simulink model "ClosedLoop_V1"  (R2021b)
settings: Solver=ode4  StartTime=0.0  StopTime=TMax  FixedStep=DT  MaxStep=DT  RelTol=1e-3  EnableMultiTasking=on
undefined symbols (not defined in the file or in its folder): CertificationSettings, Control, DiscIntNeverNeededParam, Drivetrain, OutList, P_InitAngle, RPM_Init, sigbuilder_block, SimConfig, strmatch
libraries: simulink_extras x4, simulink x1
(part 2 of 3)

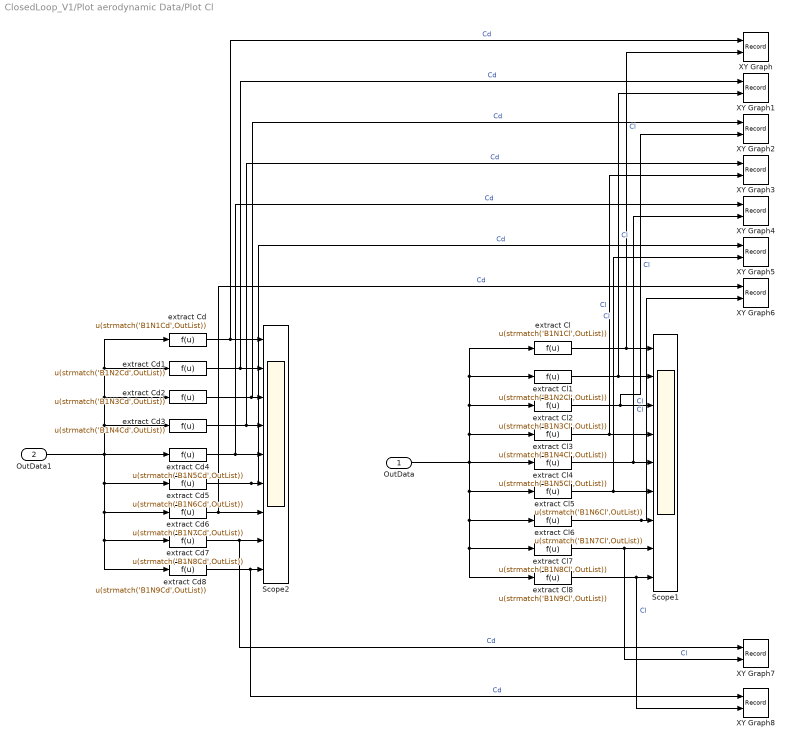
== system ClosedLoop_V1/Plot aerodynamic Data/Plot Cl ==
  OutData : Inport
  OutData1 : Inport  Port=2
  Scope1 : Scope  NumInputPorts=9
  Scope2 : Scope  NumInputPorts=9
  XY Graph : Record  FileSettingsInternal="{\"entries\":[{\"content\":{\"excelSettings\":{\"content\":{},\"type\":\"Streamout.ExcelSettings\"}},\"type\":\"Streamout.FileSettingStorage\",\"uuid\":\"b00f5487-2976-46a3-9d99-c10c1d8da87d\"}],\"packageUris\":[\"http://schema.mathworks.com/mf0/streamout_blocks/R2020a\"],\"version\":\"1.0\"}"  Layout=[1 1]  SignalsInternal="{\"entries\":[{\"content\":{\"signals\":[{\"content\":{\"blockPath\":[\"ClosedLoop_V1/Plot aerodynamic Data/Plot Cl/XY Graph\"],\"channel\":[],\"dimensions\":[1],\"domain\":\"ClosedLoop_V1/Plot aerodynamic Data/Plot Cl/XY Graph\",\"lineColor\":\"#a2142f\",\"plots\":[1],\"port\":1,\"sid\":[\"\"],\"signalID\":1325205,\"signalName\":\"Cd\"},\"type\":\"RecordBlkView.Signal\",\"uuid\":\"0eb759ee-437d-4b3f-a95d-ce2dedcb30b7\"},{\"content\":{\"blockPath\":[\"ClosedLoop_V1/Plot aerodynamic Data/Plot Cl/XY Graph\"],\"channel\":[],\"dimensions\":[1],\"domain\":\"ClosedLoop_V1/Plot aerodynamic Data/Plot Cl/XY Graph\",\"lineColor\":\"#139fff\",\"plots\":[1],\"port\":2,\"sid\":[\"\"],\"signalID\":1325209,\"signalName\":\"Cl\"},\"type\":\"RecordBlkView.Signal\",\"uuid\":\"04b02241-fa82-49a7-8999-ec9d8affa391\"}]},\"type\":\"RecordBlkView.InputSignals\",\"uuid\":\"daa39827-857a-4b2b-8609-f0bd73451858\"}],\"packageUris\":[\"http://schema.mathworks.com/mf0/streamout_blocks/R2020a\"],\"version\":\"1.0\"}"  VisualizationBindings="{\"xyplotplugin\":{\"info\":[{\"series\":[{\"bindingParametersList\":[{\"parameter\":\"X-Axis\",\"signalID\":1325205,\"signalName\":\"Cd\"},{\"parameter\":\"Y-Axis\",\"signalID\":1325209,\"signalName\":\"Cl\"}],\"seriesID\":63872}],\"subplotID\":1}]}}"  CompatibilityTag=XY  st=-1
  XY Graph1 : Record  FileSettingsInternal="{\"entries\":[{\"content\":{\"excelSettings\":{\"content\":{},\"type\":\"Streamout.ExcelSettings\"}},\"type\":\"Streamout.FileSettingStorage\",\"uuid\":\"94f4979b-c9e0-4134-9fa1-cf985e57c411\"}],\"packageUris\":[\"http://schema.mathworks.com/mf0/streamout_blocks/R2020a\"],\"version\":\"1.0\"}"  Layout=[1 1]  SignalsInternal="{\"entries\":[{\"content\":{\"signals\":[{\"content\":{\"blockPath\":[\"ClosedLoop_V1/Plot aerodynamic Data/Plot Cl/XY Graph1\"],\"channel\":[],\"dimensions\":[1],\"domain\":\"ClosedLoop_V1/Plot aerodynamic Data/Plot Cl/XY Graph1\",\"lineColor\":\"#a2142f\",\"plots\":[1],\"port\":1,\"sid\":[\"\"],\"signalID\":1325213,\"signalName\":\"Cd\"},\"type\":\"RecordBlkView.Signal\",\"uuid\":\"fcfc87ba-e672-4cf6-a8b9-8e6c01033c6e\"},{\"content\":{\"blockPath\":[\"ClosedLoop_V1/Plot aerodynamic Data/Plot Cl/XY Graph1\"],\"channel\":[],\"dimensions\":[1],\"domain\":\"ClosedLoop_V1/Plot aerodynamic Data/Plot Cl/XY Graph1\",\"lineColor\":\"#139fff\",\"plots\":[1],\"port\":2,\"sid\":[\"\"],\"signalID\":1325217,\"signalName\":\"Cl\"},\"type\":\"RecordBlkView.Signal\",\"uuid\":\"8be44a03-0071-4b23-8cb4-e834f8b4826c\"}]},\"type\":\"RecordBlkView.InputSignals\",\"uuid\":\"4f4c0f69-5f75-40c3-970b-0dcb076c4eae\"}],\"packageUris\":[\"http://schema.mathworks.com/mf0/streamout_blocks/R2020a\"],\"version\":\"1.0\"}"  VisualizationBindings="{\"xyplotplugin\":{\"info\":[{\"series\":[{\"bindingParametersList\":[{\"parameter\":\"X-Axis\",\"signalID\":1325213,\"signalName\":\"Cd\"},{\"parameter\":\"Y-Axis\",\"signalID\":1325217,\"signalName\":\"Cl\"}],\"seriesID\":24093}],\"subplotID\":1}]}}"  CompatibilityTag=XY  st=-1
  XY Graph2 : Record  FileSettingsInternal="{\"entries\":[{\"content\":{\"excelSettings\":{\"content\":{},\"type\":\"Streamout.ExcelSettings\"}},\"type\":\"Streamout.FileSettingStorage\",\"uuid\":\"4e5eaee2-b6a3-4246-9124-e66d8a1042dc\"}],\"packageUris\":[\"http://schema.mathworks.com/mf0/streamout_blocks/R2020a\"],\"version\":\"1.0\"}"  Layout=[1 1]  SignalsInternal="{\"entries\":[{\"content\":{\"signals\":[{\"content\":{\"blockPath\":[\"ClosedLoop_V1/Plot aerodynamic Data/Plot Cl/XY Graph2\"],\"channel\":[],\"dimensions\":[1],\"domain\":\"ClosedLoop_V1/Plot aerodynamic Data/Plot Cl/XY Graph2\",\"lineColor\":\"#a2142f\",\"plots\":[1],\"port\":1,\"sid\":[\"\"],\"signalID\":1325221,\"signalName\":\"Cd\"},\"type\":\"RecordBlkView.Signal\",\"uuid\":\"a1719d4d-a3ea-41e0-9451-246a2d23fc63\"},{\"content\":{\"blockPath\":[\"ClosedLoop_V1/Plot aerodynamic Data/Plot Cl/XY Graph2\"],\"channel\":[],\"dimensions\":[1],\"domain\":\"ClosedLoop_V1/Plot aerodynamic Data/Plot Cl/XY Graph2\",\"lineColor\":\"#139fff\",\"plots\":[1],\"port\":2,\"sid\":[\"\"],\"signalID\":1325225,\"signalName\":\"Cl\"},\"type\":\"RecordBlkView.Signal\",\"uuid\":\"30de273b-631d-455b-89d6-b0d743946a94\"}]},\"type\":\"RecordBlkView.InputSignals\",\"uuid\":\"fa155243-c94f-4b4c-8166-c767622a70d2\"}],\"packageUris\":[\"http://schema.mathworks.com/mf0/streamout_blocks/R2020a\"],\"version\":\"1.0\"}"  VisualizationBindings="{\"xyplotplugin\":{\"info\":[{\"series\":[{\"bindingParametersList\":[{\"parameter\":\"X-Axis\",\"signalID\":1325221,\"signalName\":\"Cd\"},{\"parameter\":\"Y-Axis\",\"signalID\":1325225,\"signalName\":\"Cl\"}],\"seriesID\":26258}],\"subplotID\":1}]}}"  CompatibilityTag=XY  st=-1
  XY Graph3 : Record  FileSettingsInternal="{\"entries\":[{\"content\":{\"excelSettings\":{\"content\":{},\"type\":\"Streamout.ExcelSettings\"}},\"type\":\"Streamout.FileSettingStorage\",\"uuid\":\"befbcad3-2241-43c1-98f9-6856619aad07\"}],\"packageUris\":[\"http://schema.mathworks.com/mf0/streamout_blocks/R2020a\"],\"version\":\"1.0\"}"  Layout=[1 1]  SignalsInternal="{\"entries\":[{\"content\":{\"signals\":[{\"content\":{\"blockPath\":[\"ClosedLoop_V1/Plot aerodynamic Data/Plot Cl/XY Graph3\"],\"channel\":[],\"dimensions\":[1],\"domain\":\"ClosedLoop_V1/Plot aerodynamic Data/Plot Cl/XY Graph3\",\"lineColor\":\"#a2142f\",\"plots\":[1],\"port\":1,\"sid\":[\"\"],\"signalID\":1325229,\"signalName\":\"Cd\"},\"type\":\"RecordBlkView.Signal\",\"uuid\":\"77f1f46a-23cf-4d3e-8ba2-b6f048b7fc30\"},{\"content\":{\"blockPath\":[\"ClosedLoop_V1/Plot aerodynamic Data/Plot Cl/XY Graph3\"],\"channel\":[],\"dimensions\":[1],\"domain\":\"ClosedLoop_V1/Plot aerodynamic Data/Plot Cl/XY Graph3\",\"lineColor\":\"#139fff\",\"plots\":[1],\"port\":2,\"sid\":[\"\"],\"signalID\":1325233,\"signalName\":\"Cl\"},\"type\":\"RecordBlkView.Signal\",\"uuid\":\"3d342543-18e3-42ba-a902-cf5380580f35\"}]},\"type\":\"RecordBlkView.InputSignals\",\"uuid\":\"aa93ef38-d005-41b7-956f-c3b12bea12ef\"}],\"packageUris\":[\"http://schema.mathworks.com/mf0/streamout_blocks/R2020a\"],\"version\":\"1.0\"}"  VisualizationBindings="{\"xyplotplugin\":{\"info\":[{\"series\":[{\"bindingParametersList\":[{\"parameter\":\"X-Axis\",\"signalID\":1325229,\"signalName\":\"Cd\"},{\"parameter\":\"Y-Axis\",\"signalID\":1325233,\"signalName\":\"Cl\"}],\"seriesID\":26014}],\"subplotID\":1}]}}"  CompatibilityTag=XY  st=-1
  XY Graph4 : Record  FileSettingsInternal="{\"entries\":[{\"content\":{\"excelSettings\":{\"content\":{},\"type\":\"Streamout.ExcelSettings\"}},\"type\":\"Streamout.FileSettingStorage\",\"uuid\":\"db6c0b38-0294-4e78-a363-89844ef9353c\"}],\"packageUris\":[\"http://schema.mathworks.com/mf0/streamout_blocks/R2020a\"],\"version\":\"1.0\"}"  Layout=[1 1]  SignalsInternal="{\"entries\":[{\"content\":{\"signals\":[{\"content\":{\"blockPath\":[\"ClosedLoop_V1/Plot aerodynamic Data/Plot Cl/XY Graph4\"],\"channel\":[],\"dimensions\":[1],\"domain\":\"ClosedLoop_V1/Plot aerodynamic Data/Plot Cl/XY Graph4\",\"lineColor\":\"#a2142f\",\"plots\":[1],\"port\":1,\"sid\":[\"\"],\"signalID\":1325237,\"signalName\":\"Cd\"},\"type\":\"RecordBlkView.Signal\",\"uuid\":\"0c91b63e-c937-4d51-adce-a1fbab03704b\"},{\"content\":{\"blockPath\":[\"ClosedLoop_V1/Plot aerodynamic Data/Plot Cl/XY Graph4\"],\"channel\":[],\"dimensions\":[1],\"domain\":\"ClosedLoop_V1/Plot aerodynamic Data/Plot Cl/XY Graph4\",\"lineColor\":\"#139fff\",\"plots\":[1],\"port\":2,\"sid\":[\"\"],\"signalID\":1325241,\"signalName\":\"Cl\"},\"type\":\"RecordBlkView.Signal\",\"uuid\":\"0b2e47cf-4e84-4860-af6a-48a2deb7a67a\"}]},\"type\":\"RecordBlkView.InputSignals\",\"uuid\":\"6ecca27e-ba54-49da-bcce-a4a3eb881ced\"}],\"packageUris\":[\"http://schema.mathworks.com/mf0/streamout_blocks/R2020a\"],\"version\":\"1.0\"}"  VisualizationBindings="{\"xyplotplugin\":{\"info\":[{\"series\":[{\"bindingParametersList\":[{\"parameter\":\"X-Axis\",\"signalID\":1325237,\"signalName\":\"Cd\"},{\"parameter\":\"Y-Axis\",\"signalID\":1325241,\"signalName\":\"Cl\"}],\"seriesID\":16519}],\"subplotID\":1}]}}"  CompatibilityTag=XY  st=-1
  XY Graph5 : Record  FileSettingsInternal="{\"entries\":[{\"content\":{\"excelSettings\":{\"content\":{},\"type\":\"Streamout.ExcelSettings\"}},\"type\":\"Streamout.FileSettingStorage\",\"uuid\":\"9460674a-7e25-40c0-b51d-5230c09c8e63\"}],\"packageUris\":[\"http://schema.mathworks.com/mf0/streamout_blocks/R2020a\"],\"version\":\"1.0\"}"  Layout=[1 1]  SignalsInternal="{\"entries\":[{\"content\":{\"signals\":[{\"content\":{\"blockPath\":[\"ClosedLoop_V1/Plot aerodynamic Data/Plot Cl/XY Graph5\"],\"channel\":[],\"dimensions\":[1],\"domain\":\"ClosedLoop_V1/Plot aerodynamic Data/Plot Cl/XY Graph5\",\"lineColor\":\"#a2142f\",\"plots\":[1],\"port\":1,\"sid\":[\"\"],\"signalID\":1325245,\"signalName\":\"Cd\"},\"type\":\"RecordBlkView.Signal\",\"uuid\":\"4c2cc2e6-f074-4467-ab2c-c656e1ab336f\"},{\"content\":{\"blockPath\":[\"ClosedLoop_V1/Plot aerodynamic Data/Plot Cl/XY Graph5\"],\"channel\":[],\"dimensions\":[1],\"domain\":\"ClosedLoop_V1/Plot aerodynamic Data/Plot Cl/XY Graph5\",\"lineColor\":\"#139fff\",\"plots\":[1],\"port\":2,\"sid\":[\"\"],\"signalID\":1325249,\"signalName\":\"Cl\"},\"type\":\"RecordBlkView.Signal\",\"uuid\":\"f16d4d46-7da3-4ca7-a621-15c7649c98ab\"}]},\"type\":\"RecordBlkView.InputSignals\",\"uuid\":\"8bb74b32-b33e-4f9b-9b24-77e9d0eb4d47\"}],\"packageUris\":[\"http://schema.mathworks.com/mf0/streamout_blocks/R2020a\"],\"version\":\"1.0\"}"  VisualizationBindings="{\"xyplotplugin\":{\"info\":[{\"series\":[{\"bindingParametersList\":[{\"parameter\":\"X-Axis\",\"signalID\":1325245,\"signalName\":\"Cd\"},{\"parameter\":\"Y-Axis\",\"signalID\":1325249,\"signalName\":\"Cl\"}],\"seriesID\":24904}],\"subplotID\":1}]}}"  CompatibilityTag=XY  st=-1
  XY Graph6 : Record  FileSettingsInternal="{\"entries\":[{\"content\":{\"excelSettings\":{\"content\":{},\"type\":\"Streamout.ExcelSettings\"}},\"type\":\"Streamout.FileSettingStorage\",\"uuid\":\"b7f41630-d128-4606-b5b0-76e3e016886f\"}],\"packageUris\":[\"http://schema.mathworks.com/mf0/streamout_blocks/R2020a\"],\"version\":\"1.0\"}"  Layout=[1 1]  SignalsInternal="{\"entries\":[{\"content\":{\"signals\":[{\"content\":{\"blockPath\":[\"ClosedLoop_V1/Plot aerodynamic Data/Plot Cl/XY Graph6\"],\"channel\":[],\"dimensions\":[1],\"domain\":\"ClosedLoop_V1/Plot aerodynamic Data/Plot Cl/XY Graph6\",\"lineColor\":\"#a2142f\",\"plots\":[1],\"port\":1,\"sid\":[\"\"],\"signalID\":1325253,\"signalName\":\"Cd\"},\"type\":\"RecordBlkView.Signal\",\"uuid\":\"3b1d38a9-1b72-4244-a152-a54677a825a9\"},{\"content\":{\"blockPath\":[\"ClosedLoop_V1/Plot aerodynamic Data/Plot Cl/XY Graph6\"],\"channel\":[],\"dimensions\":[1],\"domain\":\"ClosedLoop_V1/Plot aerodynamic Data/Plot Cl/XY Graph6\",\"lineColor\":\"#139fff\",\"plots\":[1],\"port\":2,\"sid\":[\"\"],\"signalID\":1325257,\"signalName\":\"Cl\"},\"type\":\"RecordBlkView.Signal\",\"uuid\":\"493a381b-ee0a-4854-92ec-9f5293569aef\"}]},\"type\":\"RecordBlkView.InputSignals\",\"uuid\":\"ecf3199d-e8dc-4fa5-af74-081fe56a48f2\"}],\"packageUris\":[\"http://schema.mathworks.com/mf0/streamout_blocks/R2020a\"],\"version\":\"1.0\"}"  VisualizationBindings="{\"xyplotplugin\":{\"info\":[{\"series\":[{\"bindingParametersList\":[{\"parameter\":\"X-Axis\",\"signalID\":1325253,\"signalName\":\"Cd\"},{\"parameter\":\"Y-Axis\",\"signalID\":1325257,\"signalName\":\"Cl\"}],\"seriesID\":438}],\"subplotID\":1}]}}"  CompatibilityTag=XY  st=-1
  XY Graph7 : Record  FileSettingsInternal="{\"entries\":[{\"content\":{\"excelSettings\":{\"content\":{},\"type\":\"Streamout.ExcelSettings\"}},\"type\":\"Streamout.FileSettingStorage\",\"uuid\":\"c9c28032-f02b-4770-9c4c-b7d50fb30e9d\"}],\"packageUris\":[\"http://schema.mathworks.com/mf0/streamout_blocks/R2020a\"],\"version\":\"1.0\"}"  Layout=[1 1]  SignalsInternal="{\"entries\":[{\"content\":{\"signals\":[{\"content\":{\"blockPath\":[\"ClosedLoop_V1/Plot aerodynamic Data/Plot Cl/XY Graph7\"],\"channel\":[],\"dimensions\":[1],\"domain\":\"ClosedLoop_V1/Plot aerodynamic Data/Plot Cl/XY Graph7\",\"lineColor\":\"#a2142f\",\"plots\":[1],\"port\":1,\"sid\":[\"\"],\"signalID\":1325261,\"signalName\":\"Cd\"},\"type\":\"RecordBlkView.Signal\",\"uuid\":\"4e0e9014-fb0a-41c8-a268-390f7d90f948\"},{\"content\":{\"blockPath\":[\"ClosedLoop_V1/Plot aerodynamic Data/Plot Cl/XY Graph7\"],\"channel\":[],\"dimensions\":[1],\"domain\":\"ClosedLoop_V1/Plot aerodynamic Data/Plot Cl/XY Graph7\",\"lineColor\":\"#139fff\",\"plots\":[1],\"port\":2,\"sid\":[\"\"],\"signalID\":1325265,\"signalName\":\"Cl\"},\"type\":\"RecordBlkView.Signal\",\"uuid\":\"ded6cb4d-91ec-4c24-91d7-1d6afa3da94f\"}]},\"type\":\"RecordBlkView.InputSignals\",\"uuid\":\"03fa7e92-1b0b-47ac-b291-5ef29a6e44e8\"}],\"packageUris\":[\"http://schema.mathworks.com/mf0/streamout_blocks/R2020a\"],\"version\":\"1.0\"}"  VisualizationBindings="{\"xyplotplugin\":{\"info\":[{\"series\":[{\"bindingParametersList\":[{\"parameter\":\"X-Axis\",\"signalID\":1325261,\"signalName\":\"Cd\"},{\"parameter\":\"Y-Axis\",\"signalID\":1325265,\"signalName\":\"Cl\"}],\"seriesID\":14437}],\"subplotID\":1}]}}"  CompatibilityTag=XY  st=-1
  XY Graph8 : Record  FileSettingsInternal="{\"entries\":[{\"content\":{\"excelSettings\":{\"content\":{},\"type\":\"Streamout.ExcelSettings\"}},\"type\":\"Streamout.FileSettingStorage\",\"uuid\":\"40722767-ecb4-45e0-a40b-ab64c3c9db6a\"}],\"packageUris\":[\"http://schema.mathworks.com/mf0/streamout_blocks/R2020a\"],\"version\":\"1.0\"}"  Layout=[1 1]  SignalsInternal="{\"entries\":[{\"content\":{\"signals\":[{\"content\":{\"blockPath\":[\"ClosedLoop_V1/Plot aerodynamic Data/Plot Cl/XY Graph8\"],\"channel\":[],\"dimensions\":[1],\"domain\":\"ClosedLoop_V1/Plot aerodynamic Data/Plot Cl/XY Graph8\",\"lineColor\":\"#a2142f\",\"plots\":[1],\"port\":1,\"sid\":[\"\"],\"signalID\":1325269,\"signalName\":\"Cd\"},\"type\":\"RecordBlkView.Signal\",\"uuid\":\"d84702cd-5f16-4f75-bbae-0c0931a26899\"},{\"content\":{\"blockPath\":[\"ClosedLoop_V1/Plot aerodynamic Data/Plot Cl/XY Graph8\"],\"channel\":[],\"dimensions\":[1],\"domain\":\"ClosedLoop_V1/Plot aerodynamic Data/Plot Cl/XY Graph8\",\"lineColor\":\"#139fff\",\"plots\":[1],\"port\":2,\"sid\":[\"\"],\"signalID\":1325273,\"signalName\":\"Cl\"},\"type\":\"RecordBlkView.Signal\",\"uuid\":\"e2c72b46-b8cd-45df-ac85-433b9a479b8a\"}]},\"type\":\"RecordBlkView.InputSignals\",\"uuid\":\"495dfdb2-5976-4d9a-9394-6b3494943b23\"}],\"packageUris\":[\"http://schema.mathworks.com/mf0/streamout_blocks/R2020a\"],\"version\":\"1.0\"}"  VisualizationBindings="{\"xyplotplugin\":{\"info\":[{\"series\":[{\"bindingParametersList\":[{\"parameter\":\"X-Axis\",\"signalID\":1325269,\"signalName\":\"Cd\"},{\"parameter\":\"Y-Axis\",\"signalID\":1325273,\"signalName\":\"Cl\"}],\"seriesID\":44046}],\"subplotID\":1}]}}"  CompatibilityTag=XY  st=-1
  extract Cd : Fcn  Expr=u(strmatch('B1N1Cd',OutList))
  extract Cd1 : Fcn  Expr=u(strmatch('B1N2Cd',OutList))
  extract Cd2 : Fcn  Expr=u(strmatch('B1N3Cd',OutList))
  extract Cd3 : Fcn  Expr=u(strmatch('B1N4Cd',OutList))
  extract Cd4 : Fcn  Expr=u(strmatch('B1N5Cd',OutList))
  extract Cd5 : Fcn  Expr=u(strmatch('B1N6Cd',OutList))
  extract Cd6 : Fcn  Expr=u(strmatch('B1N7Cd',OutList))
  extract Cd7 : Fcn  Expr=u(strmatch('B1N8Cd',OutList))
  extract Cd8 : Fcn  Expr=u(strmatch('B1N9Cd',OutList))
  extract Cl : Fcn  Expr=u(strmatch('B1N1Cl',OutList))
  extract Cl1 : Fcn  Expr=u(strmatch('B1N2Cl',OutList))
  extract Cl2 : Fcn  Expr=u(strmatch('B1N3Cl',OutList))
  extract Cl3 : Fcn  Expr=u(strmatch('B1N4Cl',OutList))
  extract Cl4 : Fcn  Expr=u(strmatch('B1N5Cl',OutList))
  extract Cl5 : Fcn  Expr=u(strmatch('B1N6Cl',OutList))
  extract Cl6 : Fcn  Expr=u(strmatch('B1N7Cl',OutList))
  extract Cl7 : Fcn  Expr=u(strmatch('B1N8Cl',OutList))
  extract Cl8 : Fcn  Expr=u(strmatch('B1N9Cl',OutList))
  wires:
  OutData/1 -> extract Cl/1, extract Cl1/1, extract Cl2/1, extract Cl3/1, extract Cl4/1, extract Cl5/1, extract Cl6/1, extract Cl8/1, extract Cl7/1
  extract Cl/1 -> XY Graph/2, Scope1/1  "Cl"
  extract Cl1/1 -> XY Graph1/2, Scope1/2  "Cl"
  extract Cl2/1 -> XY Graph2/2, Scope1/3  "Cl"
  extract Cl3/1 -> XY Graph3/2, Scope1/4  "Cl"
  extract Cl4/1 -> XY Graph4/2, Scope1/5  "Cl"
  extract Cl5/1 -> XY Graph5/2, Scope1/6  "Cl"
  extract Cl6/1 -> XY Graph6/2, Scope1/7  "Cl"
  extract Cl7/1 -> XY Graph7/2, Scope1/8  "Cl"
  extract Cl8/1 -> XY Graph8/2, Scope1/9  "Cl"
  extract Cd2/1 -> XY Graph2/1, Scope2/3  "Cd"
  extract Cd8/1 -> XY Graph8/1, Scope2/9  "Cd"
  extract Cd4/1 -> XY Graph4/1, Scope2/5  "Cd"
  extract Cd3/1 -> XY Graph3/1, Scope2/4  "Cd"
  extract Cd/1 -> XY Graph/1, Scope2/1  "Cd"
  OutData1/1 -> extract Cd4/1, extract Cd5/1, extract Cd6/1, extract Cd8/1, extract Cd7/1, extract Cd3/1, extract Cd2/1, extract Cd1/1, extract Cd/1
  extract Cd1/1 -> XY Graph1/1, Scope2/2  "Cd"
  extract Cd7/1 -> XY Graph7/1, Scope2/8  "Cd"
  extract Cd5/1 -> XY Graph5/1, Scope2/6  "Cd"
  extract Cd6/1 -> Scope2/7, XY Graph6/1  "Cd"

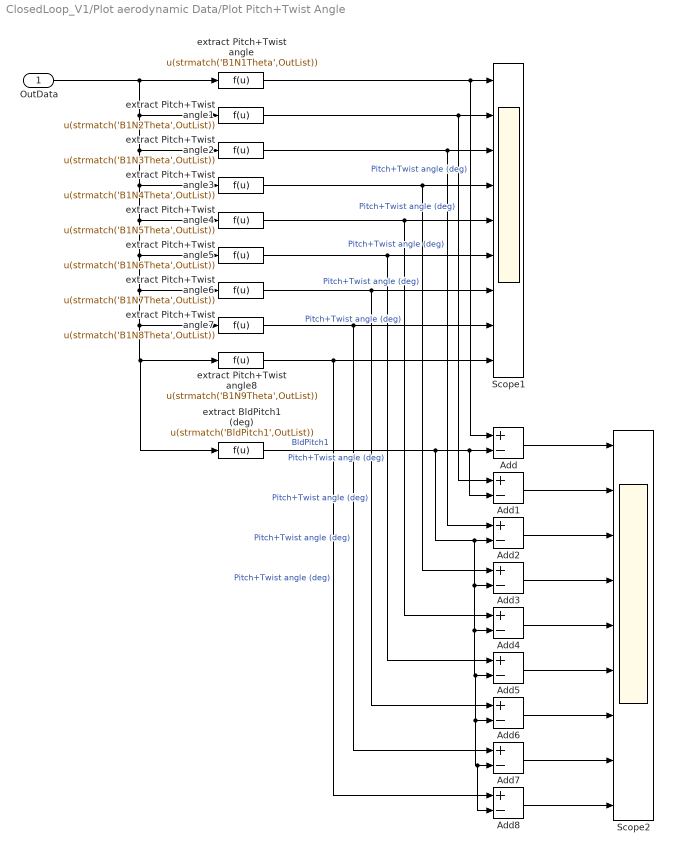
== system ClosedLoop_V1/Plot aerodynamic Data/Plot Pitch+Twist Angle ==
  OutData : Inport
  Add{,1..8} (9 alike) : Sum  Inputs=+-
  Scope1 : Scope  NumInputPorts=9
  Scope2 : Scope  NumInputPorts=9
  extract BldPitch1 (deg) : Fcn  Expr=u(strmatch('BldPitch1',OutList))
  extract Pitch+Twist angle : Fcn  Expr=u(strmatch('B1N1Theta',OutList))
  extract Pitch+Twist angle1 : Fcn  Expr=u(strmatch('B1N2Theta',OutList))
  extract Pitch+Twist angle2 : Fcn  Expr=u(strmatch('B1N3Theta',OutList))
  extract Pitch+Twist angle3 : Fcn  Expr=u(strmatch('B1N4Theta',OutList))
  extract Pitch+Twist angle4 : Fcn  Expr=u(strmatch('B1N5Theta',OutList))
  extract Pitch+Twist angle5 : Fcn  Expr=u(strmatch('B1N6Theta',OutList))
  extract Pitch+Twist angle6 : Fcn  Expr=u(strmatch('B1N7Theta',OutList))
  extract Pitch+Twist angle7 : Fcn  Expr=u(strmatch('B1N8Theta',OutList))
  extract Pitch+Twist angle8 : Fcn  Expr=u(strmatch('B1N9Theta',OutList))
  wires:
  extract Pitch+Twist angle/1 -> Add/1, Scope1/1  "Pitch+Twist angle (deg)"
  OutData/1 -> extract Pitch+Twist angle/1, extract Pitch+Twist angle1/1, extract Pitch+Twist angle2/1, extract Pitch+Twist angle3/1, extract Pitch+Twist angle4/1, extract Pitch+Twist angle5/1, extract Pitch+Twist angle6/1, extract BldPitch1 (deg)/1, extract Pitch+Twist angle8/1, extract Pitch+Twist angle7/1
  extract Pitch+Twist angle1/1 -> Add1/1, Scope1/2  "Pitch+Twist angle (deg)"
  extract Pitch+Twist angle2/1 -> Add2/1, Scope1/3  "Pitch+Twist angle (deg)"
  extract Pitch+Twist angle3/1 -> Add3/1, Scope1/4  "Pitch+Twist angle (deg)"
  extract Pitch+Twist angle4/1 -> Add4/1, Scope1/5  "Pitch+Twist angle (deg)"
  extract Pitch+Twist angle5/1 -> Add5/1, Scope1/6  "Pitch+Twist angle (deg)"
  extract Pitch+Twist angle6/1 -> Add6/1, Scope1/7  "Pitch+Twist angle (deg)"
  extract Pitch+Twist angle7/1 -> Add7/1, Scope1/8  "Pitch+Twist angle (deg)"
  extract Pitch+Twist angle8/1 -> Add8/1, Scope1/9  "Pitch+Twist angle (deg)"
  extract BldPitch1 (deg)/1 -> Add8/2, Add7/2, Add6/2, Add5/2, Add4/2, Add3/2, Add2/2, Add1/2, Add/2  "BldPitch1"
  Add/1 -> Scope2/1
  Add1/1 -> Scope2/2
  Add2/1 -> Scope2/3
  Add3/1 -> Scope2/4
  Add4/1 -> Scope2/5
  Add5/1 -> Scope2/6
  Add6/1 -> Scope2/7
  Add7/1 -> Scope2/8
  Add8/1 -> Scope2/9

== system ClosedLoop_V1/Plot aerodynamic Data/Plot Reynolds number ==
  note: B1N1Re      Reynolds number (in millions) at Blade 1, Node 1
      | B1N2Re      Reynolds number (in millions) at Blade 1, Node 2
      | B1N3Re      Reynolds number (in millions) at Blade 1, Node 3
      | B1N4Re      Reynolds number (in millions) at Blade 1, Node 4
      | B1N5Re      Reynolds number (in millions) at Blade 1, Node 5
      | B1N6Re      Reynolds number (in millions) at Blade 1, Node 6
      | B1N7Re      Reynolds number (in millions) at Blade 1, Node 7
      | B1N8Re      Reynolds number (in millions) at Blade 1, Node 8
      | B1N9Re      Reynolds number (in millions) at Blade 1, Node 9
  OutData1 : Inport
  Scope : Scope  NumInputPorts=9
  "extract Reynolds number (in millions) at Blade 1, Node 1" : Fcn  Expr=u(strmatch('B1N1Re',OutList))
  "extract Reynolds number (in millions) at Blade 1, Node 2" : Fcn  Expr=u(strmatch('B1N2Re',OutList))
  "extract Reynolds number (in millions) at Blade 1, Node 3" : Fcn  Expr=u(strmatch('B1N3Re',OutList))
  "extract Reynolds number (in millions) at Blade 1, Node 4" : Fcn  Expr=u(strmatch('B1N4Re',OutList))
  "extract Reynolds number (in millions) at Blade 1, Node 5" : Fcn  Expr=u(strmatch('B1N5Re',OutList))
  "extract Reynolds number (in millions) at Blade 1, Node 6" : Fcn  Expr=u(strmatch('B1N6Re',OutList))
  "extract Reynolds number (in millions) at Blade 1, Node 7" : Fcn  Expr=u(strmatch('B1N7Re',OutList))
  "extract Reynolds number (in millions) at Blade 1, Node 8" : Fcn  Expr=u(strmatch('B1N8Re',OutList))
  "extract Reynolds number (in millions) at Blade 1, Node 9" : Fcn  Expr=u(strmatch('B1N9Re',OutList))
  wires:
  OutData1/1 -> "extract Reynolds number (in millions) at Blade 1, Node 9"/1, "extract Reynolds number (in millions) at Blade 1, Node 8"/1, "extract Reynolds number (in millions) at Blade 1, Node 7"/1, "extract Reynolds number (in millions) at Blade 1, Node 6"/1, "extract Reynolds number (in millions) at Blade 1, Node 5"/1, "extract Reynolds number (in millions) at Blade 1, Node 4"/1, "extract Reynolds number (in millions) at Blade 1, Node 3"/1, "extract Reynolds number (in millions) at Blade 1, Node 2"/1, "extract Reynolds number (in millions) at Blade 1, Node 1"/1
  "extract Reynolds number (in millions) at Blade 1, Node 8"/1 -> Scope/8  "Reynolds number (in millions) at Blade 1, Node 8"
  "extract Reynolds number (in millions) at Blade 1, Node 3"/1 -> Scope/3  "Reynolds number (in millions) at Blade 1, Node 3"
  "extract Reynolds number (in millions) at Blade 1, Node 5"/1 -> Scope/5  "Reynolds number (in millions) at Blade 1, Node 5"
  "extract Reynolds number (in millions) at Blade 1, Node 7"/1 -> Scope/7  "Reynolds number (in millions) at Blade 1, Node 7"
  "extract Reynolds number (in millions) at Blade 1, Node 1"/1 -> Scope/1  "Reynolds number (in millions) at Blade 1, Node 1"
  "extract Reynolds number (in millions) at Blade 1, Node 6"/1 -> Scope/6  "Reynolds number (in millions) at Blade 1, Node 6"
  "extract Reynolds number (in millions) at Blade 1, Node 4"/1 -> Scope/4  "Reynolds number (in millions) at Blade 1, Node 4"
  "extract Reynolds number (in millions) at Blade 1, Node 9"/1 -> Scope/9  "Reynolds number (in millions) at Blade 1, Node 9"
  "extract Reynolds number (in millions) at Blade 1, Node 2"/1 -> Scope/2  "Reynolds number (in millions) at Blade 1, Node 2"

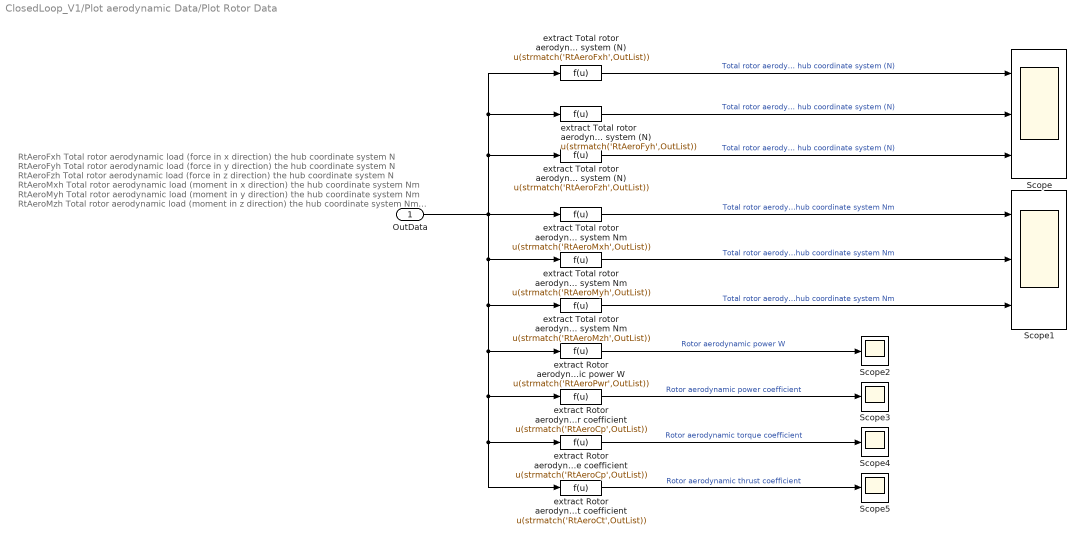
== system ClosedLoop_V1/Plot aerodynamic Data/Plot Rotor Data ==
  note: RtAeroFxh   Total rotor aerodynamic load (force in x direction) the hub coordinate system N
      | RtAeroFyh   Total rotor aerodynamic load (force in y direction) the hub coordinate system N
      | RtAeroFzh   Total rotor aerodynamic load (force in z direction) the hub coordinate system N
      | RtAeroMxh   Total rotor aerodynamic load (moment in x direction) the hub coordinate system Nm
      | RtAeroMyh   Total rotor aerodynamic load (moment in y direction) the hub coordinate system Nm
      | RtAeroMzh   Total rotor aerodynamic load (moment in z direction) the hub coordinate system Nm
      | RtAeroPwr   Rotor aerodynamic power W
      | RtAeroCp    Rotor aerodynamic power coefficient
      | RtAeroCq    Rotor aerodynamic torque coefficient
      | RtAeroCt    Rotor aerodynamic thrust coefficient
  OutData : Inport
  Scope : Scope  NumInputPorts=3
  Scope1 : Scope  NumInputPorts=3
  Scope{2..5} (4 alike) : Scope
  extract Rotor aerodynamic power W : Fcn  Expr=u(strmatch('RtAeroPwr',OutList))
  extract Rotor aerodynamic power coefficient : Fcn  Expr=u(strmatch('RtAeroCp',OutList))
  extract Rotor aerodynamic thrust coefficient : Fcn  Expr=u(strmatch('RtAeroCt',OutList))
  extract Rotor aerodynamic torque coefficient : Fcn  Expr=u(strmatch('RtAeroCp',OutList))
  extract Total rotor aerodynamic load (force in x direction) hub coordinate system (N) : Fcn  Expr=u(strmatch('RtAeroFxh',OutList))
  extract Total rotor aerodynamic load (force in y direction) hub coordinate system (N) : Fcn  Expr=u(strmatch('RtAeroFyh',OutList))
  extract Total rotor aerodynamic load (force in z direction) hub coordinate system (N) : Fcn  Expr=u(strmatch('RtAeroFzh',OutList))
  extract Total rotor aerodynamic load (moment in x direction) the hub coordinate system Nm : Fcn  Expr=u(strmatch('RtAeroMxh',OutList))
  extract Total rotor aerodynamic load (moment in y direction) the hub coordinate system Nm : Fcn  Expr=u(strmatch('RtAeroMyh',OutList))
  extract Total rotor aerodynamic load (moment in z direction) the hub coordinate system Nm : Fcn  Expr=u(strmatch('RtAeroMzh',OutList))
  wires:
  extract Total rotor aerodynamic load (force in x direction) hub coordinate system (N)/1 -> Scope/1  "Total rotor aerodynamic load (force in x direction) hub coordinate system (N)"
  OutData/1 -> extract Rotor aerodynamic thrust coefficient/1, extract Rotor aerodynamic torque coefficient/1, extract Rotor aerodynamic power coefficient/1, extract Rotor aerodynamic power W/1, extract Total rotor aerodynamic load (moment in z direction) the hub coordinate system Nm/1, extract Total rotor aerodynamic load (moment in y direction) the hub coordinate system Nm/1, extract Total rotor aerodynamic load (force in z direction) hub coordinate system (N)/1, extract Total rotor aerodynamic load (force in y direction) hub coordinate system (N)/1, extract Total rotor aerodynamic load (force in x direction) hub coordinate system (N)/1, extract Total rotor aerodynamic load (moment in x direction) the hub coordinate system Nm/1
  extract Total rotor aerodynamic load (force in y direction) hub coordinate system (N)/1 -> Scope/2  "Total rotor aerodynamic load (force in y direction) hub coordinate system (N)"
  extract Total rotor aerodynamic load (force in z direction) hub coordinate system (N)/1 -> Scope/3  "Total rotor aerodynamic load (force in z direction) hub coordinate system (N)"
  extract Total rotor aerodynamic load (moment in x direction) the hub coordinate system Nm/1 -> Scope1/1  "Total rotor aerodynamic load (moment in x direction) the hub coordinate system Nm"
  extract Total rotor aerodynamic load (moment in y direction) the hub coordinate system Nm/1 -> Scope1/2  "Total rotor aerodynamic load (moment in y direction) the hub coordinate system Nm"
  extract Total rotor aerodynamic load (moment in z direction) the hub coordinate system Nm/1 -> Scope1/3  "Total rotor aerodynamic load (moment in z direction) the hub coordinate system Nm"
  extract Rotor aerodynamic power W/1 -> Scope2/1  "Rotor aerodynamic power W"
  extract Rotor aerodynamic power coefficient/1 -> Scope3/1  "Rotor aerodynamic power coefficient"
  extract Rotor aerodynamic torque coefficient/1 -> Scope4/1  "Rotor aerodynamic torque coefficient"
  extract Rotor aerodynamic thrust coefficient/1 -> Scope5/1  "Rotor aerodynamic thrust coefficient"

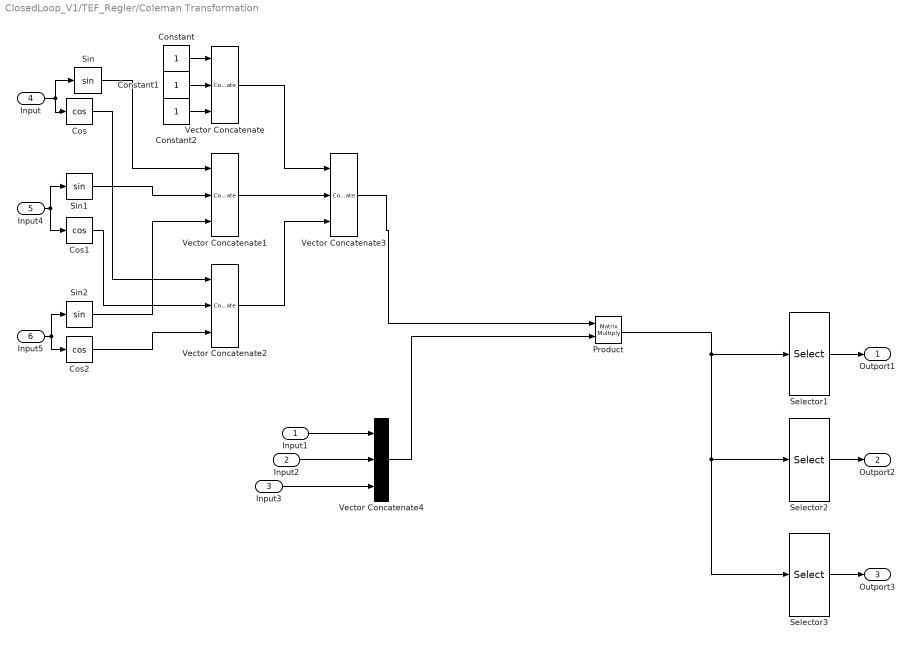
== system ClosedLoop_V1/TEF_Regler/Coleman Transformation ==
  Input1 : Inport
  Input2 : Inport  Port=2
  Input3 : Inport  Port=3
  Input : Inport  Port=4
  Input4 : Inport  Port=5
  Input5 : Inport  Port=6
  Constant : Constant
  Constant1 : Constant
  Constant2 : Constant
  Cos : Trigonometry  Operator=cos
  Cos1 : Trigonometry  Operator=cos
  Cos2 : Trigonometry  Operator=cos
  Product : Product  Multiplication=Matrix(*)
  Selector1 : Selector  InputPortWidth=3  IndexOptions=Index vector (dialog)  Indices=[1]  OutputSizes=1
  Selector2 : Selector  InputPortWidth=3  IndexOptions=Index vector (dialog)  Indices=[2]  OutputSizes=1
  Selector3 : Selector  InputPortWidth=3  IndexOptions=Index vector (dialog)  Indices=[3]  OutputSizes=1
  Sin : Trigonometry
  Sin1 : Trigonometry
  Sin2 : Trigonometry
  Vector Concatenate{,1..2,4} (4 alike) : Concatenate  NumInputs=3
  Vector Concatenate3 : Concatenate  NumInputs=3  Mode=Multidimensional array  ConcatenateDimension=2
  Outport1 : Outport  VectorParamsAs1DForOutWhenUnconnected=off
  Outport2 : Outport  Port=2  VectorParamsAs1DForOutWhenUnconnected=off
  Outport3 : Outport  Port=3  VectorParamsAs1DForOutWhenUnconnected=off
  wires:
  Vector Concatenate/1 -> Vector Concatenate3/1
  Product/1 -> Selector3/1, Selector2/1, Selector1/1
  Input/1 -> Cos/1, Sin/1
  Sin/1 -> Vector Concatenate1/1
  Cos2/1 -> Vector Concatenate2/3
  Sin1/1 -> Vector Concatenate1/2
  Cos/1 -> Vector Concatenate2/1
  Cos1/1 -> Vector Concatenate2/2
  Sin2/1 -> Vector Concatenate1/3
  Constant1/1 -> Vector Concatenate/2
  Constant/1 -> Vector Concatenate/1
  Input5/1 -> Cos2/1, Sin2/1
  Vector Concatenate1/1 -> Vector Concatenate3/2
  Vector Concatenate4/1 -> Product/2
  Selector1/1 -> Outport1/1
  Selector2/1 -> Outport2/1
  Selector3/1 -> Outport3/1
  Vector Concatenate2/1 -> Vector Concatenate3/3
  Input4/1 -> Cos1/1, Sin1/1
  Vector Concatenate3/1 -> Product/1
  Constant2/1 -> Vector Concatenate/3
  Input1/1 -> Vector Concatenate4/1
  Input2/1 -> Vector Concatenate4/2
  Input3/1 -> Vector Concatenate4/3

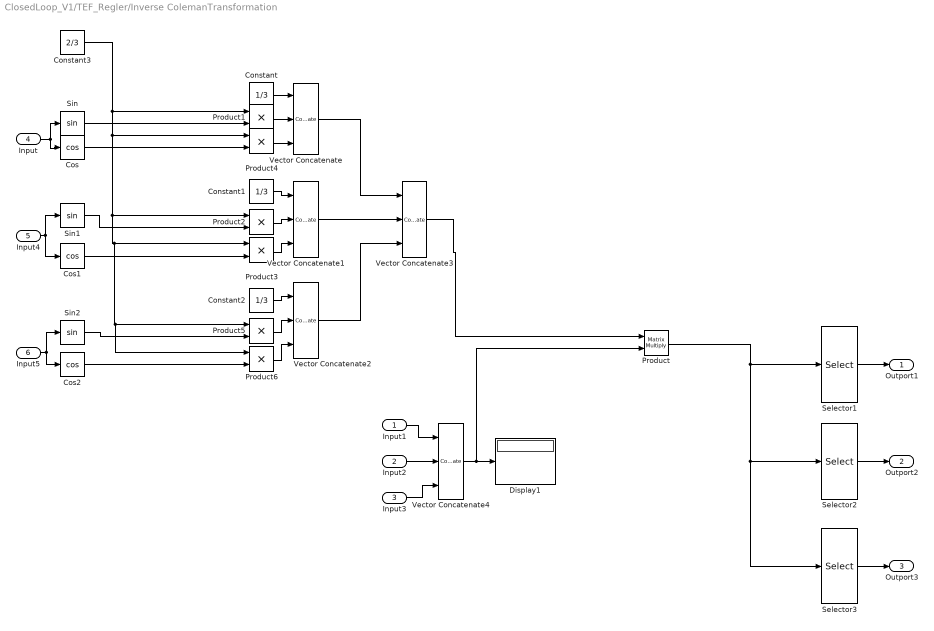
== system ClosedLoop_V1/TEF_Regler/Inverse ColemanTransformation ==
  Input1 : Inport
  Input2 : Inport  Port=2
  Input3 : Inport  Port=3
  Input : Inport  Port=4
  Input4 : Inport  Port=5
  Input5 : Inport  Port=6
  Constant : Constant  Value=1/3
  Constant1 : Constant  Value=1/3
  Constant2 : Constant  Value=1/3
  Constant3 : Constant  Value=2/3
  Cos : Trigonometry  Operator=cos
  Cos1 : Trigonometry  Operator=cos
  Cos2 : Trigonometry  Operator=cos
  Display1 : Display
  Product : Product  Multiplication=Matrix(*)
  Product{1..6} (6 alike) : Product
  Selector1 : Selector  InputPortWidth=3  IndexOptions=Index vector (dialog)  Indices=[1]  OutputSizes=1
  Selector2 : Selector  InputPortWidth=3  IndexOptions=Index vector (dialog)  Indices=[2]  OutputSizes=1
  Selector3 : Selector  InputPortWidth=3  IndexOptions=Index vector (dialog)  Indices=[3]  OutputSizes=1
  Sin : Trigonometry
  Sin1 : Trigonometry
  Sin2 : Trigonometry
  Vector Concatenate{,1..2,4} (4 alike) : Concatenate  NumInputs=3  Mode=Multidimensional array
  Vector Concatenate3 : Concatenate  NumInputs=3  Mode=Multidimensional array  ConcatenateDimension=2
  Outport1 : Outport  VectorParamsAs1DForOutWhenUnconnected=off
  Outport2 : Outport  Port=2  VectorParamsAs1DForOutWhenUnconnected=off
  Outport3 : Outport  Port=3  VectorParamsAs1DForOutWhenUnconnected=off
  wires:
  Cos2/1 -> Product6/2
  Sin2/1 -> Product5/2
  Cos1/1 -> Product3/2
  Cos/1 -> Product4/2
  Constant3/1 -> Product6/1, Product5/1, Product3/1, Product2/1, Product4/1, Product1/1
  Input2/1 -> Vector Concatenate4/2
  Input1/1 -> Vector Concatenate4/1
  Vector Concatenate4/1 -> Product/2, Display1/1
  Input3/1 -> Vector Concatenate4/3
  Product5/1 -> Vector Concatenate2/2
  Sin/1 -> Product1/2
  Product3/1 -> Vector Concatenate1/3
  Constant2/1 -> Vector Concatenate2/1
  Product6/1 -> Vector Concatenate2/3
  Constant1/1 -> Vector Concatenate1/1
  Sin1/1 -> Product2/2
  Product4/1 -> Vector Concatenate/3
  Input5/1 -> Cos2/1, Sin2/1
  Vector Concatenate3/1 -> Product/1
  Vector Concatenate/1 -> Vector Concatenate3/1
  Input/1 -> Sin/1, Cos/1
  Vector Concatenate2/1 -> Vector Concatenate3/3
  Vector Concatenate1/1 -> Vector Concatenate3/2
  Constant/1 -> Vector Concatenate/1
  Product1/1 -> Vector Concatenate/2
  Product2/1 -> Vector Concatenate1/2
  Input4/1 -> Cos1/1, Sin1/1
  Selector1/1 -> Outport1/1
  Product/1 -> Selector3/1, Selector2/1, Selector1/1
  Selector3/1 -> Outport3/1
  Selector2/1 -> Outport2/1

== system ClosedLoop_V1/TEF_Regler/Subsystem ==
  In1 : Inport
  Derivative : Derivative
  Gain : Gain  Gain=SimConfig.controller.TEF.K_P
  Gain1 : Gain  Gain=SimConfig.controller.TEF.K_I
  Gain2 : Gain  Gain=SimConfig.controller.TEF.K_D
  Integrator : Integrator
  Scope : Scope  NumInputPorts=2
  Scope1 : Scope  NumInputPorts=2
  Scope2 : Scope  NumInputPorts=5
  Sum : Sum  Inputs=+++
  Out1 : Outport  VectorParamsAs1DForOutWhenUnconnected=off
  wires:
  Sum/1 -> Scope2/4, Out1/1
  Integrator/1 -> Gain1/1  "I"
  Derivative/1 -> Gain2/1
  In1/1 -> Scope2/5, Scope/1, Gain/1, Scope1/2, Integrator/1, Derivative/1
  Gain/1 -> Scope/2, Scope2/2, Sum/2  "P"
  Gain1/1 -> Scope1/1, Scope2/3, Sum/3
  Gain2/1 -> Sum/1, Scope2/1  "D"

== system ClosedLoop_V1/TEF_Regler/Subsystem1 ==
  In1 : Inport
  Derivative : Derivative
  Gain : Gain  Gain=SimConfig.controller.TEF.K_P
  Gain1 : Gain  Gain=SimConfig.controller.TEF.K_I
  Gain2 : Gain  Gain=SimConfig.controller.TEF.K_D
  Integrator : Integrator
  Sum : Sum  Inputs=+++
  Out1 : Outport  VectorParamsAs1DForOutWhenUnconnected=off
  wires:
  Gain2/1 -> Sum/1
  Gain1/1 -> Sum/3
  Gain/1 -> Sum/2
  In1/1 -> Derivative/1, Integrator/1, Gain/1
  Derivative/1 -> Gain2/1
  Integrator/1 -> Gain1/1
  Sum/1 -> Out1/1

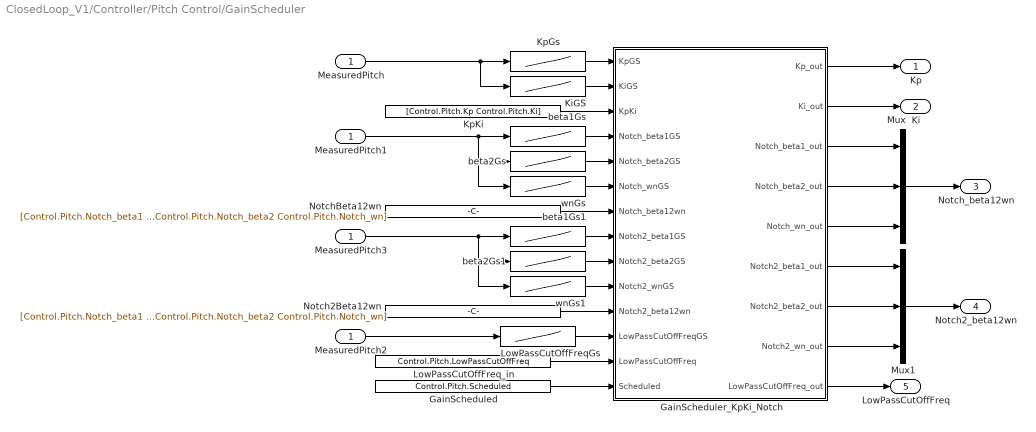
== system ClosedLoop_V1/Controller/Pitch Control/GainScheduler ==
  MeasuredPitch : Inport
  GainScheduled : Constant  Value=Control.Pitch.Scheduled
  GainScheduler_KpKi_Notch : MATLAB Function  TreatAsAtomicUnit=on
  KiGS : Lookup_n-D  NumberOfTableDimensions=1  BreakpointsForDimension1=Control.Pitch.ScheduledPitchAngles  Table=Control.Pitch.KiGS  ExtrapMethod=Clip  UseLastTableValue=on  InternalRulePriority=Speed  RndMeth=Simplest  InputSameDT=on
  KpGs : Lookup_n-D  NumberOfTableDimensions=1  BreakpointsForDimension1=Control.Pitch.ScheduledPitchAngles  Table=Control.Pitch.KpGS  ExtrapMethod=Clip  UseLastTableValue=on  InternalRulePriority=Speed  RndMeth=Simplest  InputSameDT=on
  KpKi : Constant  Value=[Control.Pitch.Kp Control.Pitch.Ki]
  LowPassCutOffFreqGs : Lookup_n-D  NumberOfTableDimensions=1  BreakpointsForDimension1=Control.Pitch.ScheduledPitchAngles  Table=Control.Pitch.LowPassCutOffFreqGS  ExtrapMethod=Clip  UseLastTableValue=on  InternalRulePriority=Speed  RndMeth=Simplest  InputSameDT=on
  LowPassCutOffFreq_in : Constant  Value=Control.Pitch.LowPassCutOffFreq
  MeasuredPitch1 : InportShadow
  MeasuredPitch2 : InportShadow
  MeasuredPitch3 : InportShadow
  Mux : Mux  Inputs=3
  Mux1 : Mux  Inputs=3
  Notch2Beta12wn : Constant  Value=[Control.Pitch.Notch_beta1 Control.Pitch.Notch_beta2 Control.Pitch.Notch_wn]
  NotchBeta12wn : Constant  Value=[Control.Pitch.Notch_beta1 Control.Pitch.Notch_beta2 Control.Pitch.Notch_wn]
  beta1Gs : Lookup_n-D  NumberOfTableDimensions=1  BreakpointsForDimension1=Control.Pitch.ScheduledPitchAngles  Table=Control.Pitch.Notch_beta1GS  ExtrapMethod=Clip  UseLastTableValue=on  InternalRulePriority=Speed  RndMeth=Simplest  InputSameDT=on
  beta1Gs1 : Lookup_n-D  NumberOfTableDimensions=1  BreakpointsForDimension1=Control.Pitch.ScheduledPitchAngles  Table=Control.Pitch.Notch2_beta1GS  ExtrapMethod=Clip  UseLastTableValue=on  InternalRulePriority=Speed  RndMeth=Simplest  InputSameDT=on
  beta2Gs : Lookup_n-D  NumberOfTableDimensions=1  BreakpointsForDimension1=Control.Pitch.ScheduledPitchAngles  Table=Control.Pitch.Notch_beta2GS  ExtrapMethod=Clip  UseLastTableValue=on  InternalRulePriority=Speed  RndMeth=Simplest  InputSameDT=on
  beta2Gs1 : Lookup_n-D  NumberOfTableDimensions=1  BreakpointsForDimension1=Control.Pitch.ScheduledPitchAngles  Table=Control.Pitch.Notch2_beta2GS  ExtrapMethod=Clip  UseLastTableValue=on  InternalRulePriority=Speed  RndMeth=Simplest  InputSameDT=on
  wnGs : Lookup_n-D  NumberOfTableDimensions=1  BreakpointsForDimension1=Control.Pitch.ScheduledPitchAngles  Table=Control.Pitch.Notch_wnGS  ExtrapMethod=Clip  UseLastTableValue=on  InternalRulePriority=Speed  RndMeth=Simplest  InputSameDT=on
  wnGs1 : Lookup_n-D  NumberOfTableDimensions=1  BreakpointsForDimension1=Control.Pitch.ScheduledPitchAngles  Table=Control.Pitch.Notch2_wnGS  ExtrapMethod=Clip  UseLastTableValue=on  InternalRulePriority=Speed  RndMeth=Simplest  InputSameDT=on
  Kp : Outport  VectorParamsAs1DForOutWhenUnconnected=off
  Ki : Outport  Port=2  VectorParamsAs1DForOutWhenUnconnected=off
  Notch_beta12wn : Outport  Port=3  VectorParamsAs1DForOutWhenUnconnected=off
  Notch2_beta12wn : Outport  Port=4  VectorParamsAs1DForOutWhenUnconnected=off
  LowPassCutOffFreq : Outport  Port=5  VectorParamsAs1DForOutWhenUnconnected=off
  wires:
  MeasuredPitch/1 -> KiGS/1, KpGs/1
  GainScheduled/1 -> GainScheduler_KpKi_Notch/14(Scheduled)
  GainScheduler_KpKi_Notch/2(Ki_out) -> Ki/1
  KpKi/1 -> GainScheduler_KpKi_Notch/3(KpKi)
  KpGs/1 -> GainScheduler_KpKi_Notch/1(KpGS)
  KiGS/1 -> GainScheduler_KpKi_Notch/2(KiGS)
  GainScheduler_KpKi_Notch/1(Kp_out) -> Kp/1
  GainScheduler_KpKi_Notch/3(Notch_beta1_out) -> Mux/1
  GainScheduler_KpKi_Notch/4(Notch_beta2_out) -> Mux/2
  GainScheduler_KpKi_Notch/5(Notch_wn_out) -> Mux/3
  NotchBeta12wn/1 -> GainScheduler_KpKi_Notch/7(Notch_beta12wn)
  MeasuredPitch1/1 -> wnGs/1, beta2Gs/1, beta1Gs/1
  beta1Gs/1 -> GainScheduler_KpKi_Notch/4(Notch_beta1GS)
  beta2Gs/1 -> GainScheduler_KpKi_Notch/5(Notch_beta2GS)
  wnGs/1 -> GainScheduler_KpKi_Notch/6(Notch_wnGS)
  Mux/1 -> Notch_beta12wn/1
  MeasuredPitch2/1 -> LowPassCutOffFreqGs/1
  LowPassCutOffFreqGs/1 -> GainScheduler_KpKi_Notch/12(LowPassCutOffFreqGS)
  LowPassCutOffFreq_in/1 -> GainScheduler_KpKi_Notch/13(LowPassCutOffFreq)
  GainScheduler_KpKi_Notch/9(LowPassCutOffFreq_out) -> LowPassCutOffFreq/1
  GainScheduler_KpKi_Notch/7(Notch2_beta2_out) -> Mux1/2
  Mux1/1 -> Notch2_beta12wn/1
  GainScheduler_KpKi_Notch/6(Notch2_beta1_out) -> Mux1/1
  GainScheduler_KpKi_Notch/8(Notch2_wn_out) -> Mux1/3
  MeasuredPitch3/1 -> wnGs1/1, beta2Gs1/1, beta1Gs1/1
  beta1Gs1/1 -> GainScheduler_KpKi_Notch/8(Notch2_beta1GS)
  beta2Gs1/1 -> GainScheduler_KpKi_Notch/9(Notch2_beta2GS)
  wnGs1/1 -> GainScheduler_KpKi_Notch/10(Notch2_wnGS)
  Notch2Beta12wn/1 -> GainScheduler_KpKi_Notch/11(Notch2_beta12wn)

== system ClosedLoop_V1/Controller/Pitch Control/Low-pass filter ==
  LowPassCutOffFreq : Inport
  u : Inport  Port=2
  Constant : Constant  Value=Control.DT
  Constant1 : Constant  Value=1/sqrt(2)
  Constant2 : Constant  Value=Control.Pitch.LowPassOrder
  Constant3 : Constant  Value=Control.DT
  First-order low-pass filter : MATLAB Function  TreatAsAtomicUnit=on
  Second-order low-pass filter : MATLAB Function  TreatAsAtomicUnit=on
  Switch : Switch  Criteria=u2 > Threshold  Threshold=1.5
  Output : Outport  VectorParamsAs1DForOutWhenUnconnected=off
  wires:
  Switch/1 -> Output/1
  Constant1/1 -> Second-order low-pass filter/3(Damp)
  Constant/1 -> Second-order low-pass filter/4(Ts)
  Constant3/1 -> First-order low-pass filter/3(Ts)
  Constant2/1 -> Switch/2
  First-order low-pass filter/1(y) -> Switch/3
  Second-order low-pass filter/1(y) -> Switch/1
  LowPassCutOffFreq/1 -> Second-order low-pass filter/2(wn), First-order low-pass filter/2(wn)
  u/1 -> First-order low-pass filter/1(u), Second-order low-pass filter/1(u)

== system ClosedLoop_V1/Controller/Pitch Control/Notch filter ==
  u : Inport
  beta12wn : Inport  Port=2
  Constant : Constant  Value=Control.DT
  Demux : Demux  Outputs=3
  MATLAB Function : MATLAB Function  TreatAsAtomicUnit=on
  Out1 : Outport  VectorParamsAs1DForOutWhenUnconnected=off
  wires:
  MATLAB Function/1(y) -> Out1/1
  Demux/1 -> MATLAB Function/2(beta1)
  Demux/2 -> MATLAB Function/3(beta2)
  Demux/3 -> MATLAB Function/4(wn)
  beta12wn/1 -> Demux/1
  u/1 -> MATLAB Function/1(u)
  Constant/1 -> MATLAB Function/5(Ts)

== system ClosedLoop_V1/Controller/Pitch Control/Notch filter1 ==
  u : Inport
  beta12wn : Inport  Port=2
  Constant : Constant  Value=Control.DT
  Demux : Demux  Outputs=3
  MATLAB Function : MATLAB Function  TreatAsAtomicUnit=on
  Out1 : Outport  VectorParamsAs1DForOutWhenUnconnected=off
  wires:
  MATLAB Function/1(y) -> Out1/1
  Demux/1 -> MATLAB Function/2(beta1)
  Demux/2 -> MATLAB Function/3(beta2)
  Demux/3 -> MATLAB Function/4(wn)
  beta12wn/1 -> Demux/1
  u/1 -> MATLAB Function/1(u)
  Constant/1 -> MATLAB Function/5(Ts)

== system ClosedLoop_V1/Controller/Torque Control/Low-pass filter ==
  u : Inport
  Constant1 : Constant  Value=Control.Torque.LowPassCutOffFreq
  Constant3 : Constant  Value=Control.DT
  First-order low-pass filter : MATLAB Function  TreatAsAtomicUnit=on
  Output : Outport  VectorParamsAs1DForOutWhenUnconnected=off
  wires:
  Constant3/1 -> First-order low-pass filter/3(Ts)
  u/1 -> First-order low-pass filter/1(u)
  First-order low-pass filter/1(y) -> Output/1
  Constant1/1 -> First-order low-pass filter/2(wn)

== matlab function ClosedLoop_V1/Controller/Pitch Control/GainScheduler/GainScheduler_KpKi_Notch ==
  data: KpGS input; KiGS input; Kp_out output; KpKi input; Notch_beta1GS input; Notch_beta2GS input; Notch_wnGS input; Notch_beta12wn input; Notch2_beta1GS input; Notch2_beta2GS input; Notch2_wnGS input; Notch2_beta12wn input; LowPassCutOffFreqGS input; LowPassCutOffFreq input; Scheduled input; Ki_out output; Notch_beta1_out output; Notch_beta2_out output; Notch_wn_out output; Notch2_beta1_out output; Notch2_beta2_out output; Notch2_wn_out output; LowPassCutOffFreq_out output
function [Kp_out, Ki_out, Notch_beta1_out, Notch_beta2_out, Notch_wn_out, Notch2_beta1_out, Notch2_beta2_out, Notch2_wn_out, LowPassCutOffFreq_out] = fcn(KpGS, KiGS, KpKi, Notch_beta1GS, Notch_beta2GS, Notch_wnGS, Notch_beta12wn, Notch2_beta1GS, Notch2_beta2GS, Notch2_wnGS, Notch2_beta12wn, LowPassCutOffFreqGS, LowPassCutOffFreq, Scheduled)

if Scheduled > 0.5
    Kp_out = KpGS;
    Ki_out = KiGS;
    Notch_beta1_out = Notch_beta1GS;
    Notch_beta2_out = Notch_beta2GS;
    Notch_wn_out = Notch_wnGS;
    Notch2_beta1_out = Notch2_beta1GS;
    Notch2_beta2_out = Notch2_beta2GS;
    Notch2_wn_out = Notch2_wnGS;
    LowPassCutOffFreq_out = LowPassCutOffFreqGS;
else
    Kp_out = KpKi(1);
    Ki_out = KpKi(2);
    Notch_beta1_out = Notch_beta12wn(1);
    Notch_beta2_out = Notch_beta12wn(2);
    Notch_wn_out = Notch_beta12wn(3);
    Notch2_beta1_out = Notch2_beta12wn(1);
    Notch2_beta2_out = Notch2_beta12wn(2);
    Notch2_wn_out = Notch2_beta12wn(3);
    LowPassCutOffFreq_out = LowPassCutOffFreq;
end

== matlab function ClosedLoop_V1/Controller/Pitch Control/Notch filter/MATLAB Function ==
  data: u input; beta1 input; beta2 input; wn input; y output; Ts input
function y = NotchFilter(u, beta1, beta2, wn, Ts)

persistent u_prev1 u_prev2 y_prev1 y_prev2
if isempty(u_prev1)
    u_prev1 = u;
    u_prev2 = u;
    y_prev1 = u;
    y_prev2 = u;
end

if any([beta1 beta2 wn] == 0)
    y = u;
else
    % Prepare filter elements from current input
    K = 2/Ts;
    Part1 = (K^2 + 2*wn*beta1 * K + wn^2) / (K^2 + 2*wn*beta2 * K + wn^2);
    Part2 = (2 * wn^2 - 2 * K^2)  / (K^2 + 2*wn*beta2 * K + wn^2);
    Part3 = (K^2 - 2*wn*beta1 * K + wn^2) / (K^2 + 2*wn*beta2 * K + wn^2);
    Part4 = (2 * wn^2 - 2 * K^2)  / (K^2 + 2*wn*beta2 * K + wn^2);
    Part5 = (K^2 - 2*wn*beta2* K + wn^2)/ (K^2 + 2*wn*beta2 * K + wn^2);
    
    % Compute filter output
    y = Part1*u + Part2*u_prev1 + Part3*u_prev2 - Part4*y_prev1 - Part5*y_prev2;
    
    % Save signals for next time step
    u_prev2 = u_prev1;
    u_prev1 = u;
    
    y_prev2 = y_prev1;
    y_prev1 = y;
end

== matlab function ClosedLoop_V1/Controller/Pitch Control/Low-pass filter/Second-order low-pass filter ==
  data: u input; wn input; Damp input; y output; Ts input
function y = SecLPF(u, wn, Damp, Ts)

persistent y_prev1 y_prev2 u_prev1 u_prev2

if isempty(u_prev1)
    y_prev1 = u;
    y_prev2 = u;
    u_prev1 = u;
    u_prev2 = u;
end

y = 1/(4+4*Ts*Damp*wn+Ts^2*wn^2) * ( (8-2*Ts^2*wn^2)*y_prev1 + ...
    (-4+4*Ts*Damp*wn-Ts^2*wn^2)*y_prev2 + (Ts^2*wn^2)*u ...
    + (2*Ts^2*wn^2)*u_prev1 + (Ts^2*wn^2)*u_prev2 );

u_prev2   = u_prev1;
u_prev1   = u;
y_prev2  = y_prev1;
y_prev1  = y;

== matlab function ClosedLoop_V1/Controller/Pitch Control/Low-pass filter/First-order low-pass filter ==
  data: u input; wn input; y output; Ts input
function y = FirstLPF(u, wn, Ts)

persistent y_prev1 u_prev1

if isempty(u_prev1)
    y_prev1 = u;
    u_prev1 = u;
end

y = (Ts*wn*u + Ts*wn*u_prev1 - (Ts*wn-2.0)*y_prev1)/(Ts*wn+2.0);

u_prev1   = u;
y_prev1  = y;

== matlab function ClosedLoop_V1/Controller/Rate Saturation Torque ==
  settings: updateMethod=DISCRETE
  data: u input; MinSaturation input; y_out output; MaxSaturation input; DT input
function y_out = fcn(u, MinSaturation, MaxSaturation, DT)
persistent y

if isempty(y)
    y = u;
end

rate = (u-y)/DT;
rate = min(max(rate, MinSaturation), MaxSaturation);

y = y + rate*DT;
y_out = y;

== matlab function ClosedLoop_V1/Controller/Pitch Control/Notch filter1/MATLAB Function ==
  data: u input; beta1 input; beta2 input; wn input; y output; Ts input
function y = NotchFilter(u, beta1, beta2, wn, Ts)

persistent u_prev1 u_prev2 y_prev1 y_prev2
if isempty(u_prev1)
    u_prev1 = u;
    u_prev2 = u;
    y_prev1 = u;
    y_prev2 = u;
end

if any([beta1 beta2 wn] == 0)
    y = u;
else
    % Prepare filter elements from current input
    K = 2/Ts;
    Part1 = (K^2 + 2*wn*beta1 * K + wn^2) / (K^2 + 2*wn*beta2 * K + wn^2);
    Part2 = (2 * wn^2 - 2 * K^2)  / (K^2 + 2*wn*beta2 * K + wn^2);
    Part3 = (K^2 - 2*wn*beta1 * K + wn^2) / (K^2 + 2*wn*beta2 * K + wn^2);
    Part4 = (2 * wn^2 - 2 * K^2)  / (K^2 + 2*wn*beta2 * K + wn^2);
    Part5 = (K^2 - 2*wn*beta2* K + wn^2)/ (K^2 + 2*wn*beta2 * K + wn^2);
    
    % Compute filter output
    y = Part1*u + Part2*u_prev1 + Part3*u_prev2 - Part4*y_prev1 - Part5*y_prev2;
    
    % Save signals for next time step
    u_prev2 = u_prev1;
    u_prev1 = u;
    
    y_prev2 = y_prev1;
    y_prev1 = y;
end

== matlab function ClosedLoop_V1/Controller/Torque Control/Low-pass filter/First-order low-pass filter ==
  data: u input; wn input; y output; Ts input
function y = FirstLPF(u, wn, Ts)

persistent y_prev1 u_prev1

if isempty(u_prev1)
    y_prev1 = u;
    u_prev1 = u;
end

y = (Ts*wn*u + Ts*wn*u_prev1 - (Ts*wn-2.0)*y_prev1)/(Ts*wn+2.0);

u_prev1   = u;
y_prev1  = y;

== matlab function ClosedLoop_V1/Controller/Torque Control/TorqueController ==
  data: GeneratorTorqueDemand output; MeasuredGeneratorSpeed input; MeasuredPitch input; Control_Torque_OptGain input; omega_ABCD input size=[1 4]; P_StartupMode input; Torque_Demanded input; FineMaxPitch input; T_MinTorque input; Clock input; Event input; EventTime input
function GeneratorTorqueDemand  = TorqueController(MeasuredGeneratorSpeed, MeasuredPitch, Control_Torque_OptGain, omega_ABCD, P_StartupMode, Torque_Demanded, FineMaxPitch, T_MinTorque, Clock, Event, EventTime)

% Calculate generator torque setpoint according to the feedforward wind
% turbine control law T = K*\omega^2
GeneratorTorqueDemand = max(min(Control_Torque_OptGain*MeasuredGeneratorSpeed^2, Torque_Demanded), T_MinTorque);

% Calculate torques at beginning and end of CP_max operation
TorqueOmegaB = Control_Torque_OptGain*(omega_ABCD(2)*pi/30)^2;
TorqueOmegaC = Control_Torque_OptGain*(omega_ABCD(3)*pi/30)^2;

% Apply maximum demanded torque when pitch is 1 degree above fine-pitch and
% the wind turbine is not in start-up mode.
if (Event == 5 && Clock >= EventTime) && (MeasuredPitch > (FineMaxPitch(2) - 1.0)*pi/180) %Emergency shutdown
    GeneratorTorqueDemand = 0.0;
elseif MeasuredPitch > (FineMaxPitch(1) + 1.0)*pi/180 && P_StartupMode == false
    GeneratorTorqueDemand = Torque_Demanded;
elseif MeasuredGeneratorSpeed < omega_ABCD(1)*pi/30
    GeneratorTorqueDemand = T_MinTorque;
elseif MeasuredGeneratorSpeed < omega_ABCD(2)*pi/30
    GeneratorTorqueDemand = (TorqueOmegaB - T_MinTorque)/((omega_ABCD(2) - omega_ABCD(1))*pi/30)*(MeasuredGeneratorSpeed - omega_ABCD(1)*pi/30) + T_MinTorque;
elseif MeasuredGeneratorSpeed >= omega_ABCD(3)*pi/30
    GeneratorTorqueDemand = (Torque_Demanded - TorqueOmegaC)/((omega_ABCD(4) - omega_ABCD(3))*pi/30)*(MeasuredGeneratorSpeed - omega_ABCD(3)*pi/30) + TorqueOmegaC;
end

== matlab function ClosedLoop_V1/MATLAB Function2 ==
  data: switch_signal input; Output output; Input_1 input; Input_2 input
function Output  = fcn(switch_signal, Input_1, Input_2)

if switch_signal == 1
    Output = Input_1;
else
    Output = Input_2;
end

== matlab function ClosedLoop_V1/Individual Pitch Controller/MATLAB Function ==
  data: M1 input; M_N2 output; M2 input; M3 input; Phi input; M_N3 output
function [M_N2, M_N3] = fcn(M1,M2,M3,Phi)

M_N2 = 2/3 * cos(Phi) * M1 + 2/3 * cos(Phi+2*pi/3) * M2 + 2/3 * cos(Phi+4*pi/3) * M3;
M_N3 = 2/3 * sin(Phi) * M1 + 2/3 * sin(Phi+2*pi/3) * M2 + 2/3 * sin(Phi+4*pi/3) * M3;

== matlab function ClosedLoop_V1/Individual Pitch Controller/MATLAB Function1 ==
  data: M_N2 input; beta output; M_N3 input; Phi input
function beta  = fcn(M_N2,M_N3,Phi)

beta_1 = cos(Phi) * M_N2 + sin(Phi) * M_N3;
beta_2 = cos(Phi+2*pi/3) * M_N2 + sin(Phi+2*pi/3) * M_N3;
beta_3 = cos(Phi+4*pi/3) * M_N2 + sin(Phi+4*pi/3) * M_N3;

beta = [beta_1,beta_2,beta_3];

== matlab function ClosedLoop_V1/Individual Pitch Controller/Rate Saturation Pitch ==
  settings: updateMethod=DISCRETE
  data: u input; MinSaturation input; y_out output; MaxSaturation input; DT input
function y_out = fcn(u, MinSaturation, MaxSaturation, DT)
persistent y

if isempty(y)
    y = u;
end

rate = (u-y)/DT;
rate = min(max(rate, MinSaturation), MaxSaturation);

y = y + rate*DT;
y_out = y;

== matlab function ClosedLoop_V1/MATLAB Function3 ==
  data: switch_signal input; Output output; Input_1 input; Input_2 input
function Output  = fcn(switch_signal, Input_1, Input_2)

if switch_signal == 1
    Output = Input_1;
else
    Output = Input_2;
end
